simulink model "Water_tank_lab1"  (R2022a)
settings: Solver=VariableStepAuto  StartTime=0.0  StopTime=1000  RelTol=1e-3
libraries: slpidlib x1
settings Model: Creator=eriks  LastModifiedBy=eriks

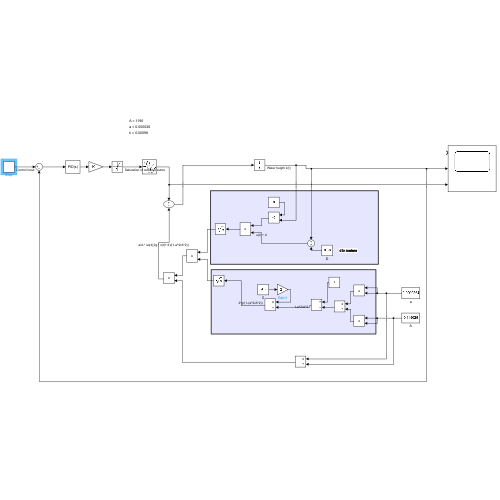
[thumbnail: Simulink's stored preview of the top-level diagram]
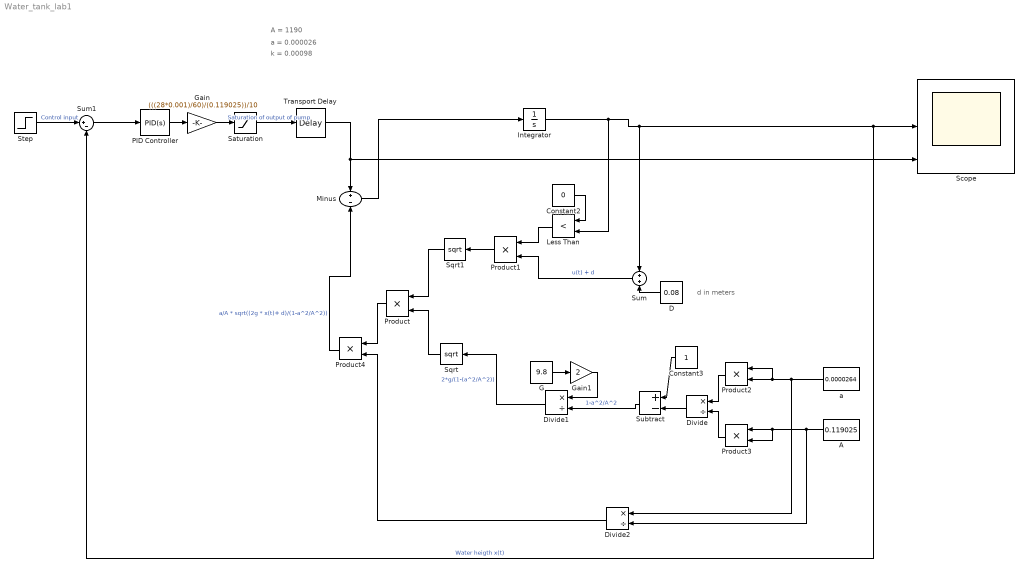
== system Water_tank_lab1 ==
  note: A = 1190
  note: k = 0.00098
  note: a = 0.000026
  note: d in meters
  A : Constant  Value=0.119025
  Constant2 : Constant  Value=0
  Constant3 : Constant
  D : Constant  Value=0.08
  Divide : Product  Inputs=*/
  Divide1 : Product  Inputs=*/
  Divide2 : Product  Inputs=*/
  G : Constant  Value=9.8
  Gain : Gain  Gain=(((28*0.001)/60)/(0.119025))/10
  Gain1 : Gain  Gain=2
  Integrator : Integrator  InitialCondition=0.535
  Less Than : RelationalOperator  Operator=<  OutDataTypeStr=boolean  RndMeth=Simplest  InputSameDT=off
  Minus : Sum  Inputs=+-
  PID Controller : slpidlib/PID Controller  Controller=PID  Form=Parallel  TimeDomain=Continuous-time  UseExternalTs=off  SampleTime=-1  IntegratorMethod=Forward Euler  FilterMethod=Forward Euler  ControllerParametersSource=internal  P=1  I=1  UseKiTs=off  D=0  N=100  UseFilter=on  TunerSelectOption=Frequency Response Based  InitialConditionSource=internal  InitialConditionForIntegrator=0  InitialConditionForFilter=0  DifferentiatorICPrevScaledInput=0  ExternalReset=none  TrackingMode=off  Kt=1  LimitOutput=off  SatLimitsSource=internal  UpperSaturationLimit=inf  LowerSaturationLimit=-inf  LinearizeAsGain=on  AntiWindupMode=none  Kb=1  POutMin=[]  POutMax=[]  IOutMin=[]  IOutMax=[]  DOutMin=[]  DOutMax=[]  NOutMin=[]  NOutMax=[]  SumOutMin=[]  SumOutMax=[]  SaturationOutMin=[]  SaturationOutMax=[]  PParamMin=[]  PParamMax=[]  IParamMin=[]  IParamMax=[]  DParamMin=[]  DParamMax=[]  NParamMin=[]  NParamMax=[]  KbParamMin=[]  KbParamMax=[]  KtParamMin=[]  KtParamMax=[]  KbOutMin=[]  KbOutMax=[]  KtOutMin=[]  KtOutMax=[]  IntegratorOutMin=[]  IntegratorOutMax=[]  FilterOutMin=[]  FilterOutMax=[]  SumI1OutMin=[]  SumI1OutMax=[]  SumI2OutMin=[]  SumI2OutMax=[]  SumI3OutMin=[]  SumI3OutMax=[]  SumI4OutMin=[]  SumI4OutMax=[]  SumDOutMin=[]  SumDOutMax=[]  DifferentiatorOutMin=[]  DifferentiatorOutMax=[]  FilterDiffOutCoefMin=[]  FilterDiffOutCoefMax=[]  ReciprocalOutMin=[]  ReciprocalOutMax=[]  SumDenOutMin=[]  SumDenOutMax=[]  SumNumOutMin=[]  SumNumOutMax=[]  DivideOutMin=[]  DivideOutMax=[]  UdiffTsProdOutMin=[]  UdiffTsProdOutMax=[]  NTsProdOutMin=[]  NTsProdOutMax=[]  UintegralTsProdOutMin=[]  UintegralTsProdOutMax=[]  UngainTsProdOutMin=[]  UngainTsProdOutMax=[]  IntegratorContinuousStateAttributes=''  IntegratorStateMustResolveToSignalObject=off  IntegratorRTWStateStorageClass=Auto  FilterContinuousStateAttributes=''  FilterStateMustResolveToSignalObject=off  FilterRTWStateStorageClass=Auto  ParallelPVariant=InternalParameters  IdealPVariant=Disabled  IVariant=InternalParameters  DVariant=InternalParameters  IntegratorVariant=Continuous  SatVariant=Disabled  AWVariant=Passthrough  PCopyVariant=Disabled  TRVariant=Disabled  FdbkBlocksVariant=Forward  IdealPFdbkVariant=Disabled  SatFdbkVariant=Disabled  DerivativeFilterVariant=ContFilter  NVariant=InternalParameters  NCopyVariant=Disabled  FilterICVariant=InternalICsFilter  IntegratorICVariant=InternalICs  ExternalResetVariant=Disabled  TRSumVariant=Passthrough  SumFdbkVariant=Disabled  SumVariant=Sum_PID  TsampFilterVariant=InternalTs  TsampNgainVariant=Passthrough  TsampIntegralVariant=Passthrough  ExternalSaturationOutDataTypeStr=Inherit: Same as second input  aMode=0
  Product{,1..4} (5 alike) : Product
  Saturation : Saturate  UpperLimit=((28*0.001)/60)/0.119025  LowerLimit=0
  Scope : Scope  NumInputPorts=3
  Sqrt : Sqrt
  Sqrt1 : Sqrt
  Step : Step  After=0.64  SampleTime=0
  Subtract : Sum  Inputs=+-
  Sum : Sum
  Sum1 : Sum  Inputs=|+-
  Transport Delay : TransportDelay  DelayTime=315
  a : Constant  Value=0.0000264
  wires:
  Integrator/1 -> Less Than/2, Sum/1, Scope/2, Sum1/2  "Water heigth x(t)"
  D/1 -> Sum/2
  Sqrt/1 -> Product/2
  Minus/1 -> Integrator/1
  Sum/1 -> Product1/2  "u(t) + d"
  a/1 -> Product2/2, Product2/1, Divide2/1
  A/1 -> Product3/1, Product3/2, Divide2/2
  Divide/1 -> Subtract/2
  Constant3/1 -> Subtract/1
  Subtract/1 -> Divide1/2  "1-a^2/A^2"
  Saturation/1 -> Transport Delay/1  "Saturation of output of pump"
  Product2/1 -> Divide/1
  Product3/1 -> Divide/2
  G/1 -> Gain1/1
  Divide2/1 -> Product4/2
  Product4/1 -> Minus/2  "a/A * sqrt((2g * x(t)+ d)/(1-a^2/A^2))"
  Constant2/1 -> Less Than/1
  Less Than/1 -> Product1/1
  Product1/1 -> Sqrt1/1
  Divide1/1 -> Sqrt/1  "2*g/(1-(a^2/A^2))"
  Sqrt1/1 -> Product/1
  Product/1 -> Product4/1
  Gain/1 -> Saturation/1
  Transport Delay/1 -> Scope/3, Minus/1
  PID Controller/1 -> Gain/1
  Gain1/1 -> Divide1/1
  Sum1/1 -> PID Controller/1
  Step/1 -> Sum1/1  "Control input"
